simulink model "mech_flexible_four_bar"  (Simulink 7.1)
settings: Solver=ode23t  StartTime=0.0  StopTime=10.0  AbsTol=5e-3
PreLoadFcn:
  | %-----------------------------------------
  | % Defined in the block mask
  | %-----------------------------------------
  | fBeamElement.material = 'Mild Steel';
  | 
  | % Beam element density (Kg/m^3)
  | fBeamElement.density = 7600;
  | 
  | fBeamElement.LengX = 1E-2;
  | fBeamElement.LengY = 1E-2;
  | 
  | % Beam element area of cross-section (m^2)
  | fBeamElement.crossArea = fBeamElement.LengX * fBeamElement.LengY;
  | 
  | % Beam element length (m)
  | fBeamElement.length = 0.2;
  | 
  | % Length of CG vector along length of beam (m)
  | fBeamElement.cgLeng = fBeamElement.length/2;
  | 
  | % Beam element direction (along X direction it is [1 0 0])
  | fBeamElement.beamDir = [0 1 0];
  | 
  | % Beam element Mass Moment of Inertia (Kg/m^2)
  | fBeamElement.Inertia = [6400.0 0 0;0 120 0;0 0 6400.0]*5E-8;
  | 
  | % Beam element Youngs Modulus (N/m^2)
  | fBeamElement.youngsM = 100E8;
  | 
  | % Beam element Shear Modulus (N/m^2)
  | fBeamElement.shearM = 26E9;
  | 
  | % Beam element Area Moment of Inertia along the direction of bending (m^4)
  | fBeamElement.Ixx = fBeamElement.LengX * fBeamElement.LengY^3/12;
  | 
  | % Beam element Area Moment of Inertia normal to the direction of
  | % bending (m^4)
  | fBeamElement.Iyy = fBeamElement.LengY * fBeamElement.LengX^3/12;
  | 
  | % Damping Coeff
  | fBeamElement.matDamping = 2;
  | %-----------------------------------------
InitFcn:
  | %-----------------------------------------
  | % Defined in the block mask
  | %-----------------------------------------
  | fBeamElement.material = 'Mild Steel';
  | 
  | % Beam element density (Kg/m^3)
  | fBeamElement.density = 7600;
  | 
  | fBeamElement.LengX = 1E-2;
  | fBeamElement.LengY = 1E-2;
  | 
  | % Beam element area of cross-section (m^2)
  | fBeamElement.crossArea = fBeamElement.LengX * fBeamElement.LengY;
  | 
  | % Beam element length (m)
  | fBeamElement.length = 0.2;
  | 
  | % Length of CG vector along length of beam (m)
  | fBeamElement.cgLeng = fBeamElement.length/2;
  | 
  | % Beam element direction (along X direction it is [1 0 0])
  | fBeamElement.beamDir = [0 1 0];
  | 
  | % Beam element Mass Moment of Inertia (Kg/m^2)
  | fBeamElement.Inertia = [6400.0 0 0;0 120 0;0 0 6400.0]*5E-8;
  | 
  | % Beam element Youngs Modulus (N/m^2)
  | fBeamElement.youngsM = 100E8;
  | 
  | % Beam element Shear Modulus (N/m^2)
  | fBeamElement.shearM = 26E9;
  | 
  | % Beam element Area Moment of Inertia along the direction of bending (m^4)
  | fBeamElement.Ixx = fBeamElement.LengX * fBeamElement.LengY^3/12;
  | 
  | % Beam element Area Moment of Inertia normal to the direction of
  | % bending (m^4)
  | fBeamElement.Iyy = fBeamElement.LengY * fBeamElement.LengX^3/12;
  | 
  | % Damping Coeff
  | fBeamElement.matDamping = 2;
  | %-----------------------------------------
libraries: mblibv1 x12, mech_flexible_element_lib x5
Description:
  | Flexible Four Bar Mechanism
  | 
  | Closed-loop machine with one flexible bar turning under the influence of gravity.
settings Model: Creator=arnav  LastModifiedBy=batserve  ExtModeAutoUpdateStatusClock=off
settings SolverCC: InsertRTBMode=Auto
settings DataIOCC: SignalLoggingName=sigsOut  OutputTimes=linspace(0,10,500);
settings OptimizationCC: BooleanDataType=off  InlineInvariantSignals=on
settings DebuggingCC: SaveWithParameterizedLinksMsg=none  CheckExecutionContextPreStartOutputMsg=on  CheckExecutionContextRuntimeOutputMsg=on  SignalResolutionControl=TryResolveAllWithWarning  SolverPrmCheckMsg=none  MultiTaskDSMMsg=warning  MultiTaskCondExecSysMsg=none  SigSpecEnsureSampleTimeMsg=none  UnconnectedInputMsg=none  UnconnectedOutputMsg=none  UnconnectedLineMsg=none  StrictBusMsg=None
settings HardwareCC: TargetBitPerLong=64  TargetEndianess=LittleEndian  TargetWordSize=64  TargetHWDeviceType=MATLAB Host  ProdEqTarget=off
settings RTWCC: SystemTargetFile=rsim.tlc  TemplateMakefile=rsim_default_tmf  Description=Rapid Simulation Target  ProcessScript=rsim_make_rtw_hook  IncludeERTFirstTime=on
settings RSimTargetCC: TargetFcnLib=ansi_tfl_tmw.mat  TargetFunctionLibrary=ANSI_C  IsPILTarget=off  EnableShiftOperators=on  PortableWordSizes=off
settings SimMechanicsCC: WarnOnRedundantConstraints=off  VisOnUpdateDiagram=on

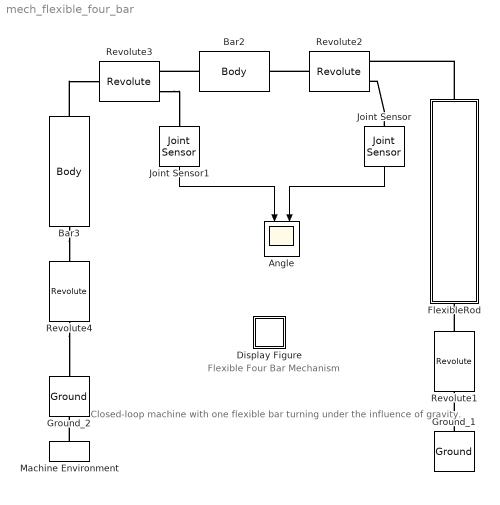
== system mech_flexible_four_bar ==
  note: Flexible Four Bar Mechanism
  note: Closed-loop machine with one flexible
      | bar turning under the influence of gravity.
  Angle : Scope  NumInputPorts=2
      settings: Orientation=down  TimeRange=0.1  YMin=-17.5~2.5  YMax=-14~3.1
  Bar2 : mblibv1/Bodies/Body  Orientation=left  DialogController=MECH.DynMechDlgSource  PhysicalDomain=mechanical  SubClassName=Unknown  LeftPortType=workingframe  RightPortType=workingframe  LConnTagsString=CS1  RConnTagsString=CS2  DialogClass=MechanicalBodyBlock  Mass=9.028  MassUnits=kg  InertiaUnits=kg*m^2  Inertia=[1.8e-3 0 0;0 0.678 0;0 0 0.678]  Shape=Cylinder  ShapeDims=[1 1]  ShapeUnits=m  ShapeUse=false  Density=1  DensityUnits=kg/m^3  DensityUse=false  GraphicsMode=1  BodyColor=[0.5 0.5 0.5]  GraphicsObj=[]  AttachedToCS=1  CG=Left$CG$[-0.427 -0.242 0]$WORLD$CS1$m$[0 0 29.5]$Euler X-Y-Z$deg$WORLD$false  WorkingFrames=Left$CS1$[0 0 0]$WORLD$ADJOINING$m$[0 0 0]$Euler X-Y-Z$deg$WORLD$true#Right$CS2$[-0.87 -0.493 0]$WORLD$CS1$m$[0 0 0]$Euler X-Y-Z$deg$WORLD$true  CGPos=[-0.427 -0.242 0]  CGRot=[0 0 29.5]  CS0Pos=[]  CS0Rot=[]  CS1Pos=[0 0 0]  CS1Rot=[0 0 0]  CS2Pos=[-0.87 -0.493 0]  CS2Rot=[0 0 0]  CS3Pos=[]  CS3Rot=[]  CS4Pos=[]  CS4Rot=[]  CS5Pos=[]  CS5Rot=[]  CS6Pos=[]  CS6Rot=[]  CS7Pos=[]  CS7Rot=[]  CS8Pos=[]  CS8Rot=[]  CS9Pos=[]  CS9Rot=[]  CS10Pos=[]  CS10Rot=[]  CS11Pos=[]  CS11Rot=[]  CS12Pos=[]  CS12Rot=[]  CS13Pos=[]  CS13Rot=[]  CS14Pos=[]  CS14Rot=[]  CS15Pos=[]  CS15Rot=[]  CS16Pos=[]  CS16Rot=[]  CS17Pos=[]  CS17Rot=[]  CS18Pos=[]  CS18Rot=[]  CS19Pos=[]  CS19Rot=[]  CS20Pos=[]  CS20Rot=[]
  Bar3 : mblibv1/Bodies/Body  Orientation=down  DialogController=MECH.DynMechDlgSource  PhysicalDomain=mechanical  SubClassName=Unknown  LeftPortType=workingframe  RightPortType=workingframe  LConnTagsString=CS1  RConnTagsString=CS2  DialogClass=MechanicalBodyBlock  Mass=0.5  MassUnits=kg  InertiaUnits=kg*m^2  Inertia=[1.0e-5 0 0;0 1.1e-3 0;0 0 1.1e-3]*5  Shape=Cylinder  ShapeDims=[1 1]  ShapeUnits=m  ShapeUse=false  Density=1  DensityUnits=kg/m^3  DensityUse=false  GraphicsMode=1  BodyColor=[0.5 0.5 0.5]  GraphicsObj=[]  AttachedToCS=1  CG=Left$CG$[-0.03 -0.25 0]$WORLD$CS1$m$[0 0 93]$Euler X-Y-Z$deg$WORLD$false  WorkingFrames=Left$CS1$[0 0 0]$WORLD$ADJOINING$m$[0 0 0]$Euler X-Y-Z$deg$WORLD$true#Right$CS2$[0 0 0]$WORLD$ADJOINING$m$[0 0 0]$Euler X-Y-Z$deg$WORLD$true  CGPos=[-0.03 -0.25 0]  CGRot=[0 0 93]  CS0Pos=[]  CS0Rot=[]  CS1Pos=[0 0 0]  CS1Rot=[0 0 0]  CS2Pos=[0 0 0]  CS2Rot=[0 0 0]  CS3Pos=[]  CS3Rot=[]  CS4Pos=[]  CS4Rot=[]  CS5Pos=[]  CS5Rot=[]  CS6Pos=[]  CS6Rot=[]  CS7Pos=[]  CS7Rot=[]  CS8Pos=[]  CS8Rot=[]  CS9Pos=[]  CS9Rot=[]  CS10Pos=[]  CS10Rot=[]  CS11Pos=[]  CS11Rot=[]  CS12Pos=[]  CS12Rot=[]  CS13Pos=[]  CS13Rot=[]  CS14Pos=[]  CS14Rot=[]  CS15Pos=[]  CS15Rot=[]  CS16Pos=[]  CS16Rot=[]  CS17Pos=[]  CS17Rot=[]  CS18Pos=[]  CS18Rot=[]  CS19Pos=[]  CS19Rot=[]  CS20Pos=[]  CS20Rot=[]
  Display Figure : Subsystem  Tag=Help  Description="Help callback for four bar model: mech_four_bar.  Opens Help browser to Type 19 marker at documentation for this tutorial model."
      settings: OpenFcn=helpview([docroot '/toolbox/physmod/mech/mech.map'], 'mech_four_bar_help');
      mask Type: Help callback
      mask Display: image(imread('info.bmp'))
  FlexibleRod : Subsystem  Orientation=up
  Ground_1 : mblibv1/Bodies/Ground  Orientation=up  DialogController=MECH.DynMechDlgSource  SystemSampleTime=-1  LeftPortType=env  RightPortType=workingframe  PhysicalDomain=Mechanical  DialogClass=GroundBlock  CoordPosition=[0.433 0.04 0]  CoordPositionUnits=m  StateVectorMgrId=-1  MachineId=[0 0]  ShowEnvPort=off
  Ground_2 : mblibv1/Bodies/Ground  Orientation=up  DialogController=MECH.DynMechDlgSource  SystemSampleTime=-1  LeftPortType=env  RightPortType=workingframe  PhysicalDomain=Mechanical  DialogClass=GroundBlock  CoordPosition=[-0.434 0.04 0]  CoordPositionUnits=m  StateVectorMgrId=-1  MachineId=[0 0]  ShowEnvPort=on
  Joint Sensor : mblibv1/Sensors &  Actuators/Joint Sensor  Orientation=down  DialogController=MECH.DynMechDlgSource  SystemSampleTime=-1  PhysicalDomain=Mechanical  PortType=blob  Muxed=on  Pose=on  Angle=on  AngleUnits=deg  ArcVelocity=off  ArcVelocityUnits=deg/s  ArcAcceleration=off  ArcAccelerationUnits=deg/s^2  CoordPosition=on  CoordPositionUnits=m  Velocity=off  VelocityUnits=m/s  Acceleration=off  AccelerationUnits=m/s^2  Quaternion=on  QuaternionDT=off  QuaternionDDT=off  QuaternionUnits=off  OutputVector=[1]  ActiveIO=on  Width=1  DialogClass=MechanicalSensorBlock  Primitive=R1  Force=off  ForceUnits=N  Torque=off  TorqueUnits=N-m  ReferenceFrame=Absolute (INERTIAL)  ReactionSensedSide=Base  ReactionReferenceFrame=Absolute (World)  ReactionForce=off  ReactionForceUnits=N  ReactionMoment=off  ReactionMomentUnits=N-m
  Joint Sensor1 : mblibv1/Sensors &  Actuators/Joint Sensor  Orientation=down  DialogController=MECH.DynMechDlgSource  SystemSampleTime=-1  PhysicalDomain=Mechanical  PortType=blob  Muxed=on  Pose=on  Angle=on  AngleUnits=deg  ArcVelocity=off  ArcVelocityUnits=deg/s  ArcAcceleration=off  ArcAccelerationUnits=deg/s^2  CoordPosition=on  CoordPositionUnits=m  Velocity=off  VelocityUnits=m/s  Acceleration=off  AccelerationUnits=m/s^2  Quaternion=on  QuaternionDT=off  QuaternionDDT=off  QuaternionUnits=off  OutputVector=[1]  ActiveIO=on  Width=1  DialogClass=MechanicalSensorBlock  Primitive=R1  Force=off  ForceUnits=N  Torque=off  TorqueUnits=N-m  ReferenceFrame=Absolute (INERTIAL)  ReactionSensedSide=Base  ReactionReferenceFrame=Absolute (World)  ReactionForce=off  ReactionForceUnits=N  ReactionMoment=off  ReactionMomentUnits=N-m
  Machine Environment : mblibv1/Bodies/Machine Environment  Tag=Factory ground  Orientation=up  DialogController=MECH.DialogSource  SystemSampleTime=-1  PortType=env  PhysicalDomain=Mechanical  DialogTemplateClass=MECH.MachineEnvironment  SyncWhenCopied=off  Gravity=[0 -9.81 0]  GravityUnits=m/s^2  GravityAsSignal=off  Dimensionality=3D Only  AnalysisType=Forward dynamics  LinearAssemblyTolerance=1e-3  LinearAssemblyToleranceUnits=m  AngularAssemblyTolerance=1e-3  AngularAssemblyToleranceUnits=rad  ConstraintSolverType=Stabilizing  ConstraintRelTolerance=1e-4  ConstraintAbsTolerance=1e-4  UseRobustSingularityHandling=off  RedundancyAnalysisToleranceType=Automatically select tolerance  RedundancyAnalysisTolerance=1e-14  StatePerturbationType=Adaptive  PerturbationSize=1e-3  VisualizeMachine=on
  Revolute1 : mblibv1/Joints/Revolute  Orientation=down  DialogController=MECH.DynMechDlgSource  PhysicalDomain=mechanical  SubClassName=Unknown  LeftPortType=blob  RightPortType=blob  LConnTagsString=__newl0  RConnTagsString=__newr0  NumSAPorts=0  CutJoint=off  MarkAsCut=off  Primitives=revolute  PrimitiveProps=R1$WORLD$[0 0 1]$revolute  DialogClass=JointBlock  R1Axis=[0 0 1]
  Revolute2 : mblibv1/Joints/Revolute  Orientation=left  DialogController=MECH.DynMechDlgSource  PhysicalDomain=mechanical  SubClassName=Unknown  LeftPortType=blob  RightPortType=blob  LConnTagsString=__newl0|SA1  RConnTagsString=__newr0  NumSAPorts=1  CutJoint=off  MarkAsCut=off  Primitives=revolute  PrimitiveProps=R1$WORLD$[0 0 1]$revolute  DialogClass=JointBlock  R1Axis=[0 0 1]
  Revolute3 : mblibv1/Joints/Revolute  Orientation=left  DialogController=MECH.DynMechDlgSource  PhysicalDomain=mechanical  SubClassName=Unknown  LeftPortType=blob  RightPortType=blob  LConnTagsString=__newl0|SA1  RConnTagsString=__newr0  NumSAPorts=1  CutJoint=off  MarkAsCut=off  Primitives=revolute  PrimitiveProps=R1$WORLD$[0 0 1]$revolute  DialogClass=JointBlock  R1Axis=[0 0 1]
  Revolute4 : mblibv1/Joints/Revolute  Orientation=down  DialogController=MECH.DynMechDlgSource  PhysicalDomain=mechanical  SubClassName=Unknown  LeftPortType=blob  RightPortType=blob  LConnTagsString=__newl0  RConnTagsString=__newr0  NumSAPorts=0  CutJoint=off  MarkAsCut=off  Primitives=revolute  PrimitiveProps=R1$WORLD$[0 0 1]$revolute  DialogClass=JointBlock  R1Axis=[0 0 1]
  wires:
  Joint Sensor1/1 -> Angle/1
  Joint Sensor/1 -> Angle/2
  connections:
  Joint Sensor/LConn1 -- Revolute2/LConn2
  FlexibleRod/RConn1 -- Revolute2/LConn1
  Revolute2/RConn1 -- Bar2/LConn1
  Bar2/RConn1 -- Revolute3/LConn1
  Bar3/LConn1 -- Revolute3/RConn1
  Bar3/RConn1 -- Revolute4/LConn1
  Revolute3/LConn2 -- Joint Sensor1/LConn1
  Revolute4/RConn1 -- Ground_2/RConn1
  Machine Environment/RConn1 -- Ground_2/LConn1
  Ground_1/RConn1 -- Revolute1/RConn1
  Revolute1/LConn1 -- FlexibleRod/LConn1

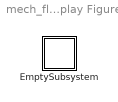
== system mech_flexible_four_bar/Display Figure ==
  EmptySubsystem : Subsystem

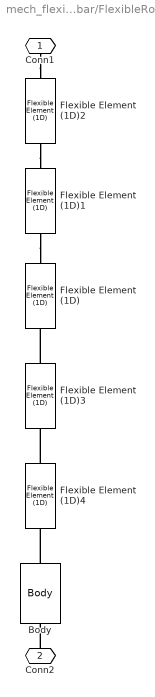
== system mech_flexible_four_bar/FlexibleRod ==
  Body : mblibv1/Bodies/Body  Orientation=up  DialogController=MECH.DynMechDlgSource  PhysicalDomain=mechanical  SubClassName=Unknown  LeftPortType=workingframe  RightPortType=workingframe  LConnTagsString=CS1  RConnTagsString=CS2  DialogClass=MechanicalBodyBlock  Mass=1  MassUnits=kg  InertiaUnits=kg*m^2  Inertia=eye(3)*1E-8  Shape=Cylinder  ShapeDims=[1 1]  ShapeUnits=m  ShapeUse=false  Density=1  DensityUnits=kg/m^3  DensityUse=false  GraphicsMode=1  BodyColor=[0.5 0.5 0.5]  GraphicsObj=[]  AttachedToCS=1  CG=Left$CG$[0 0 0]$CS1$CS1$m$[0 0 0]$Euler X-Y-Z$deg$WORLD$false  WorkingFrames=Left$CS1$[0 0 0]$ADJOINING$ADJOINING$m$[0 0 0]$Euler X-Y-Z$deg$WORLD$true#Right$CS2$[0 0 0]$CS1$CS1$m$[0 0 0]$Euler X-Y-Z$deg$WORLD$true  CGPos=[0 0 0]  CGRot=[0 0 0]  CS0Pos=[]  CS0Rot=[]  CS1Pos=[0 0 0]  CS1Rot=[0 0 0]  CS2Pos=[0 0 0]  CS2Rot=[0 0 0]  CS3Pos=[]  CS3Rot=[]  CS4Pos=[]  CS4Rot=[]  CS5Pos=[]  CS5Rot=[]  CS6Pos=[]  CS6Rot=[]  CS7Pos=[]  CS7Rot=[]  CS8Pos=[]  CS8Rot=[]  CS9Pos=[]  CS9Rot=[]  CS10Pos=[]  CS10Rot=[]  CS11Pos=[]  CS11Rot=[]  CS12Pos=[]  CS12Rot=[]  CS13Pos=[]  CS13Rot=[]  CS14Pos=[]  CS14Rot=[]  CS15Pos=[]  CS15Rot=[]  CS16Pos=[]  CS16Rot=[]  CS17Pos=[]  CS17Rot=[]  CS18Pos=[]  CS18Rot=[]  CS19Pos=[]  CS19Rot=[]  CS20Pos=[]  CS20Rot=[]
  Flexible Element (1D){,1..4} (5 alike) : mech_flexible_element_lib/Flexible Element (1D)  Orientation=up  SystemSampleTime=-1  material=Mild Steel  density=fBeamElement.density  crossArea=fBeamElement.crossArea  length=fBeamElement.length  cgLeng=fBeamElement.cgLeng  beamDir=fBeamElement.beamDir  Inertia=fBeamElement.Inertia  youngsM=fBeamElement.youngsM  shearM=26E9  Ixx=fBeamElement.Ixx  Iyy=8.3333e-010  matDamping=fBeamElement.matDamping
  Conn1 : PMIOPort  Orientation=down  Port=1  Side=Right
  Conn2 : PMIOPort  Orientation=up  Port=2  Side=Left
  connections:
  Flexible Element (1D)1/LConn1 -- Flexible Element (1D)/RConn1
  Flexible Element (1D)2/LConn1 -- Flexible Element (1D)1/RConn1
  Conn1/RConn1 -- Flexible Element (1D)2/RConn1
  Conn2/RConn1 -- Body/LConn1
  Body/RConn1 -- Flexible Element (1D)4/LConn1
  Flexible Element (1D)4/RConn1 -- Flexible Element (1D)3/LConn1
  Flexible Element (1D)3/RConn1 -- Flexible Element (1D)/LConn1

== system mech_flexible_four_bar/Display Figure/EmptySubsystem ==
